simulink model "HysteresisTestStub"  (R2020a)
settings: Solver=FixedStepAuto  StartTime=0.0  StopTime=10.0  FixedStep=1e-3  RelTol=1e-3  EnableMultiTasking=on
settings Model: ExtModeTrigDuration=5  Creator=liams  LastModifiedBy=liams
settings OptimizationCC: EnhancedBackFolding=on  PassReuseOutputArgsAs=Individual arguments  ZeroExternalMemoryAtStartup=off  ZeroInternalMemoryAtStartup=off  MaxStackSize=64  OptimizeBlockOrder=speed  DifferentSizesBufferReuse=on  OptimizationCustomize=off  EfficientTunableParamExpr=on
settings DebuggingCC: ParameterTunabilityLossMsg=error
settings HardwareCC: ProdBitPerPointer=32  ProdBitPerSizeT=32  ProdBitPerPtrDiffT=32  ProdLargestAtomicInteger=Long  ProdLargestAtomicFloat=Double  ProdWordSize=32  ProdHWDeviceType=ARM Compatible->ARM Cortex
settings SFSimCC: MATLABDynamicMemAlloc=off
settings RTWCC: SystemTargetFile=ert.tlc  HardwareBoard=NXP FRDM-K64F  TemplateMakefile=ert_default_tmf  Toolchain=GNU Tools for ARM Embedded Processors
settings CodeAppCC: ForceParamTrailComments=on  IgnoreCustomStorageClasses=off  OperatorAnnotations=on  SimulinkDataObjDesc=on  SFDataObjDesc=on  InsertBlockDesc=on

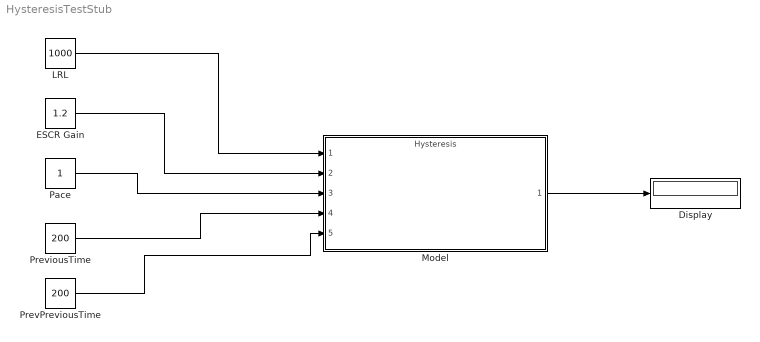
== system HysteresisTestStub ==
  Display : Display
  ESCR Gain : Constant  Value=1.2
  LRL : Constant  Value=1000
  Model : ModelReference  ModelNameDialog=Hysteresis.slx  SimulationMode=Normal  ModelReferenceVersion=1.2
  Pace : Constant  OutDataTypeStr=boolean
  PrevPreviousTime : Constant  Value=200
  PreviousTime : Constant  Value=200
  wires:
  LRL/1 -> Model/1
  ESCR Gain/1 -> Model/2
  Pace/1 -> Model/3
  PreviousTime/1 -> Model/4
  PrevPreviousTime/1 -> Model/5
  Model/1 -> Display/1
